simulink model "gazebo_uav"  (R2019b)
settings: Solver=VariableStepAuto  StartTime=0.0  StopTime=10  RelTol=1e-3
undefined symbols (not defined in the file): body, duration, force_type, fx, fy, fz, iris, link_name, model_name, torque_type, tx, ty, tz
libraries: robotgazebolib x5, robotcorelib x1
settings Model: Creator=darrahts  LastModifiedBy=darrahts

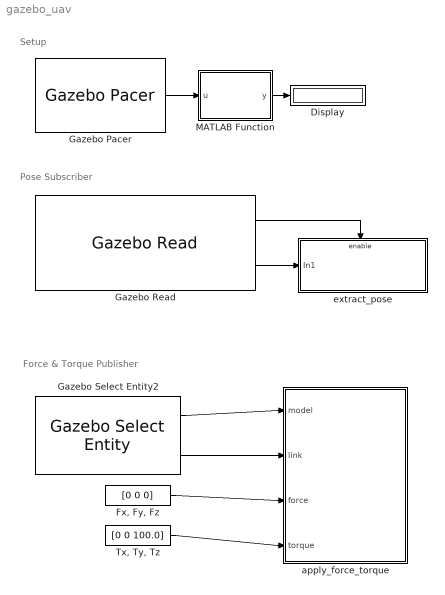
== system gazebo_uav ==
  note: Setup
  note: Pose Subscriber
  note: Force & Torque Publisher
  Display : Display
  "Fx, Fy, Fz" : Constant  Value=[0 0 0]
  Gazebo Pacer : robotgazebolib/Gazebo Pacer  ResetBehavior=Reset Gazebo simulation time and scene  SampleTime=0.01
      settings: SourceProductName=Robotics System Toolbox  SourceProductBaseCode=RO
  Gazebo Read : robotgazebolib/Gazebo Read  topicSource=From Gazebo  topic=/gazebo/ground_truth/world_pose/iris/base_link  messageType=gazebo_msgs/Pose  sampleTime=.01
      settings: SourceProductName=Robotics System Toolbox  SourceProductBaseCode=RO
  Gazebo Select Entity2 : robotgazebolib/Gazebo Select Entity  modelElemName=iris/body  outputArraySize=128  OutputLabel=Link  SelectType=Link
      settings: SourceProductName=Robotics System Toolbox  SourceProductBaseCode=RO
  MATLAB Function : MATLAB Function  TreatAsAtomicUnit=on
  "Tx, Ty, Tz" : Constant  Value=[0 0 100.0]
  apply_force_torque : Subsystem
  extract_pose : Subsystem
  wires:
  Gazebo Pacer/1 -> MATLAB Function/1(u)
  Gazebo Read/1 -> extract_pose/Enable
  Gazebo Read/2 -> extract_pose/1(In1)
  MATLAB Function/1(y) -> Display/1
  Gazebo Select Entity2/2 -> apply_force_torque/2(link)
  Gazebo Select Entity2/1 -> apply_force_torque/1(model)
  "Fx, Fy, Fz"/1 -> apply_force_torque/3(force)
  "Tx, Ty, Tz"/1 -> apply_force_torque/4(torque)

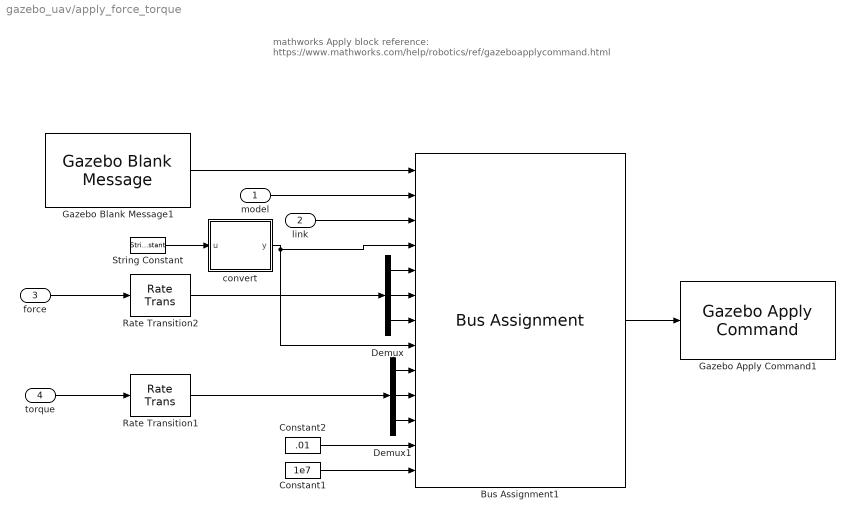
== system gazebo_uav/apply_force_torque ==
  note: mathworks Apply block reference: https://www.mathworks.com/help/robotics/ref/gazeboapplycommand.html
  model : Inport
  link : Inport  Port=2
  force : Inport  Port=3
  torque : Inport  Port=4
  Bus Assignment1 : BusAssignment  AssignedSignals=model_name,link_name,force_type,fx,fy,fz,torque_type,tx,ty,tz,duration.seconds,duration.nano_seconds
  Constant1 : Constant  Value=1e7
  Constant2 : Constant  Value=.01
  Demux : Demux  Outputs=3
  Demux1 : Demux  Outputs=3
  Gazebo Apply Command1 : robotgazebolib/Gazebo Apply Command  cmdType=ApplyLinkWrench  sampleTime=0.01
      settings: SourceProductName=Robotics System Toolbox  SourceProductBaseCode=RO
  Gazebo Blank Message1 : robotgazebolib/Gazebo Blank Message  msgType=ApplyLinkWrench  sampleTime=0.01  busName='Gazebo_SL_Bus_gazebo_msgs_ApplyLinkWrench'
      settings: SourceProductName=Robotics System Toolbox  SourceProductBaseCode=RO
  Rate Transition1 : RateTransition
  Rate Transition2 : RateTransition
  String Constant : StringConstant  String="\"SET\""
  convert : MATLAB Function  TreatAsAtomicUnit=on
  wires:
  Rate Transition2/1 -> Demux/1
  Gazebo Blank Message1/1 -> Bus Assignment1/1
  Bus Assignment1/1 -> Gazebo Apply Command1/1
  force/1 -> Rate Transition2/1
  model/1 -> Bus Assignment1/2
  link/1 -> Bus Assignment1/3
  String Constant/1 -> convert/1(u)
  Constant2/1 -> Bus Assignment1/12
  Demux/3 -> Bus Assignment1/7
  Demux/2 -> Bus Assignment1/6
  Demux/1 -> Bus Assignment1/5
  Demux1/2 -> Bus Assignment1/10
  torque/1 -> Rate Transition1/1
  Demux1/3 -> Bus Assignment1/11
  Demux1/1 -> Bus Assignment1/9
  Rate Transition1/1 -> Demux1/1
  convert/1(y) -> Bus Assignment1/8, Bus Assignment1/4
  Constant1/1 -> Bus Assignment1/13

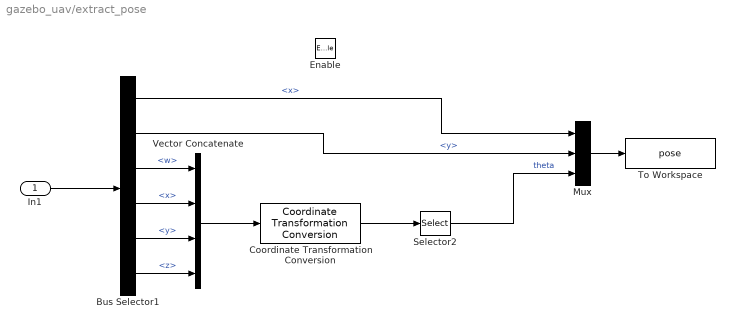
== system gazebo_uav/extract_pose ==
  In1 : Inport
  Enable : EnablePort
  Bus Selector1 : BusSelector  OutputSignals=position.x,position.y,orientation.w,orientation.x,orientation.y,orientation.z
  Coordinate Transformation Conversion : robotcorelib/Coordinate Transformation Conversion  InputRepresentation=Quaternion  InputEulerSequence=ZYX  ShowTrVecInputPort=on  OutputRepresentation=Euler Angles  OutputEulerSequence=ZYX  ShowTrVecOutputPort=on  SimulateUsing=Interpreted execution
      settings: SourceProductBaseCode=RO
  Mux : Mux  Inputs=3
  Selector2 : Selector  InputPortWidth=3  IndexOptions=Index vector (dialog)  Indices=1  OutputSizes=1
  To Workspace : ToWorkspace  VariableName=pose  SaveFormat=Timeseries  SampleTime=-1
  Vector Concatenate : Concatenate  NumInputs=4
  wires:
  Vector Concatenate/1 -> Coordinate Transformation Conversion/1
  Coordinate Transformation Conversion/1 -> Selector2/1
  Selector2/1 -> Mux/3  "theta"
  Bus Selector1/6 -> Vector Concatenate/4  "<z>"
  Bus Selector1/4 -> Vector Concatenate/2  "<x>"
  Bus Selector1/3 -> Vector Concatenate/1  "<w>"
  Bus Selector1/5 -> Vector Concatenate/3  "<y>"
  In1/1 -> Bus Selector1/1
  Bus Selector1/1 -> Mux/1  "<x>"
  Bus Selector1/2 -> Mux/2  "<y>"
  Mux/1 -> To Workspace/1

== matlab function gazebo_uav/MATLAB Function ==
  data: u input; y output
function y = assert(u)

    if u == 0
        y = "synchronized";
    else
        y = "error";
    end

== matlab function gazebo_uav/apply_force_torque/convert ==
  data: u input; y output size=128
function y = convert(u)

y = uint8(convertStringsToChars(u))';
